simulink model "model_response_zmp12"  (Simulink 7.9)
settings: Solver=ode45  StartTime=0.0  StopTime=10.0  RelTol=1e-3
undefined symbols (not defined in the file or in its folder): kp
settings Model: Creator=pajon  LastModifiedBy=pajon

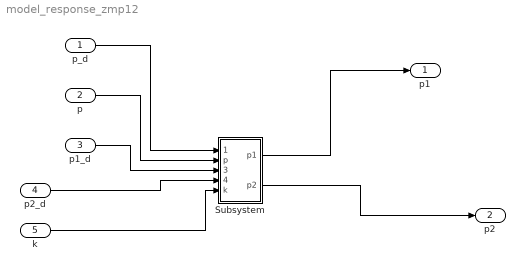
== system model_response_zmp12 ==
  p_d : Inport
  p : Inport  Port=2
  p1_d : Inport  Port=3
  p2_d : Inport  Port=4
  k : Inport  Port=5
  Subsystem : Subsystem
  p1 : Outport
  p2 : Outport  Port=2
  wires:
  p_d/1 -> Subsystem/1(p_d)
  Subsystem/1(p1) -> p1/1
  p/1 -> Subsystem/2(p)
  p1_d/1 -> Subsystem/3(p1_d)
  Subsystem/2(p2) -> p2/1
  p2_d/1 -> Subsystem/4(p2_d)
  k/1 -> Subsystem/5(k)

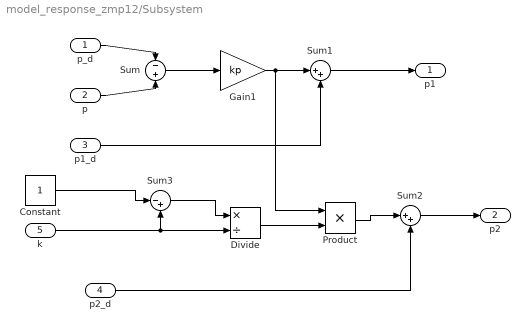
== system model_response_zmp12/Subsystem ==
  p_d : Inport
  p : Inport  Port=2
  p1_d : Inport  Port=3
  p2_d : Inport  Port=4
  k : Inport  Port=5
  Constant : Constant
  Divide : Product  Inputs=*/
  Gain1 : Gain  Gain=kp
  Product : Product  RndMeth=Zero
  Sum : Sum  Inputs=-+
  Sum1 : Sum  Inputs=|++
  Sum2 : Sum  Inputs=|++
  Sum3 : Sum  Inputs=|-+
  p1 : Outport
  p2 : Outport  Port=2
  wires:
  p_d/1 -> Sum/1
  p/1 -> Sum/2
  Sum/1 -> Gain1/1
  Gain1/1 -> Sum1/1, Product/1
  p1_d/1 -> Sum1/2
  Sum1/1 -> p1/1
  p2_d/1 -> Sum2/2
  Sum2/1 -> p2/1
  k/1 -> Divide/2, Sum3/2
  Sum3/1 -> Divide/1
  Constant/1 -> Sum3/1
  Product/1 -> Sum2/1
  Divide/1 -> Product/2
